simulink model "hover"  (R2021a)
settings: Solver=VariableStepAuto  StartTime=0.0  StopTime=10.0  RelTol=1e-3
model workspace (MAT data in the model file):
  A = [0  0  0  0  1  0  0  0; 0  0  0  0  0  1  0  0; 0  0  0  0  0  0  1  0; 0  0  0  0  0  0  0  1; 0  0  0  0  0  0  0  0; 0  0  0  0  0  0  0  0; 0  0  0  0  0  0  0  0; 0  0  0  0  0  0  0  0]
  B = [0  0  0  0; 0  0  0  0; 0  0  0  0; 0  0  0  0; -0.000322580645161  0  0  0; 0  0.005  0  0; 0  0  0.001  0; 0  0  0  0.000666666666667]
  Bf = [1  1  1  1  1  1  1  1  1  1  1  1; 4  3  2  -2  -3  -4  4  3  2  -2  -3  -4; 2.1  2.1  2.1  2.1  2.1  2.1  -3.9  -3.9  -3.9  -3.9  -3.9  -3.9; -0.1  -0.1  -0.1  0.1  0.1  0.1  -0.1  -0.1  -0.1  0.1  0.1  0.1]
  G = [30400.615; 0; 0; 0]
  Jf = [-3100  0  0  0; 0  200  0  0; 0  0  1000  0; 0  0  0  1500]
  Jx = 200
  Jy = 1000
  Jz = 1500
  eta_rot = [1 1 1 1 1 1 1 1 1 1 1 1]
  g = 9.80665
  k_mu = 0.1
  m = 3100
  w_rot = [-1 -1 -1 1 1 1 -1 -1 -1 1 1 1]
  x_cg = -2.6
  x_rot = [-0.5 -0.5 -0.5 -0.5 -0.5 -0.5 -6.5 -6.5 -6.5 -6.5 -6.5 -6.5]
  y_cg = 0
  y_rot = [-4 -3 -2 2 3 4 -4 -3 -2 2 3 4]
settings Model: Creator=jakob  LastModifiedBy=jakob

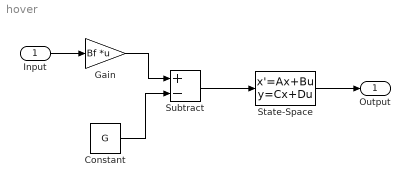
== system hover ==
  Input : Inport
  Constant : Constant  Value=G
  Gain : Gain  Gain=Bf  Multiplication=Matrix(K*u)
  State-Space : StateSpace  A=A  B=B  C=eye(8)  D=zeros(8, 4)  InitialCondition=zeros(8,1)
  Subtract : Sum  Inputs=+-
  Output : Outport
  wires:
  Subtract/1 -> State-Space/1
  Constant/1 -> Subtract/2
  Gain/1 -> Subtract/1
  Input/1 -> Gain/1
  State-Space/1 -> Output/1
